simulink model "PID_centerlineTracking"  (R2023b)
settings: Solver=VariableStepAuto  StartTime=0.0  StopTime=Te  RelTol=1e-3
values from neighbouring files (symbols this model uses):
  Ts = 0.1    [ScriptBoot.m]    (also in ScriptBoot_TEST.m)
undefined symbols (not defined in the file or in its folder): accMAX, brakeMAX, driving, egoCarID, jerkMAX, lr, m, position0, turnAngleMAX, turnAngleRateMAX, velocity0
libraries: drivingscenarioandsensors x7, robotcorelib x2, autolibshared x1, sensorinslib x1
(part 1 of 3)
settings Model: Creator=Victor  LastModifiedBy=Victor

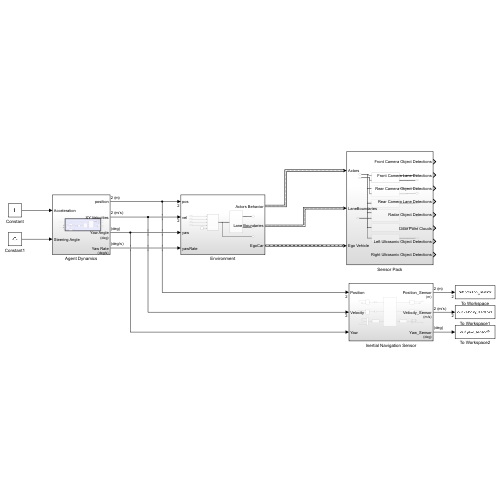
[thumbnail: Simulink's stored preview of the top-level diagram]
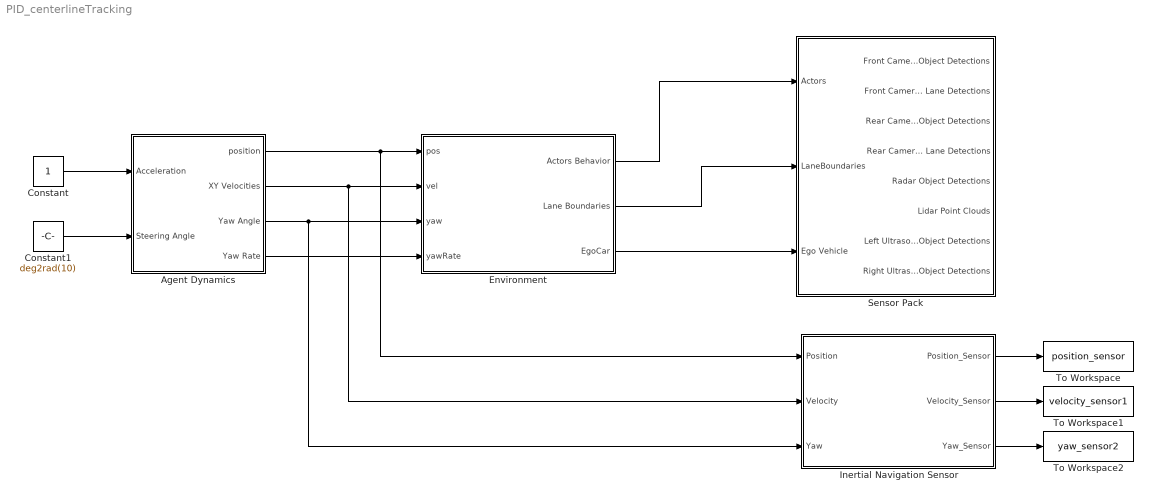
== system PID_centerlineTracking ==
  Agent Dynamics : Subsystem
  Constant : Constant
  Constant1 : Constant  Value=deg2rad(10)
  Environment : Subsystem
  Inertial Navigation Sensor : Subsystem
  Sensor Pack : Subsystem
  To Workspace : ToWorkspace  VariableName=position_sensor  SaveFormat=Timeseries  SampleTime=-1
  To Workspace1 : ToWorkspace  VariableName=velocity_sensor1  SaveFormat=Timeseries  SampleTime=-1
  To Workspace2 : ToWorkspace  VariableName=yaw_sensor2  SaveFormat=Timeseries  SampleTime=-1
  wires:
  Constant/1 -> Agent Dynamics/1(Acceleration)
  Constant1/1 -> Agent Dynamics/2(Steering Angle)
  Agent Dynamics/1(position) -> Inertial Navigation Sensor/1(Position), Environment/1(pos)
  Agent Dynamics/2(XY Velocities) -> Inertial Navigation Sensor/2(Velocity), Environment/2(vel)
  Agent Dynamics/3(Yaw Angle) -> Inertial Navigation Sensor/3(Yaw), Environment/3(yaw)
  Agent Dynamics/4(Yaw Rate) -> Environment/4(yawRate)
  Inertial Navigation Sensor/3(Yaw_Sensor) -> To Workspace2/1
  Inertial Navigation Sensor/2(Velocity_Sensor) -> To Workspace1/1
  Inertial Navigation Sensor/1(Position_Sensor) -> To Workspace/1
  Environment/1(Actors Behavior) -> Sensor Pack/1(Actors)
  Environment/2(Lane Boundaries) -> Sensor Pack/2(LaneBoundaries)
  Environment/3(EgoCar) -> Sensor Pack/3(Ego Vehicle)

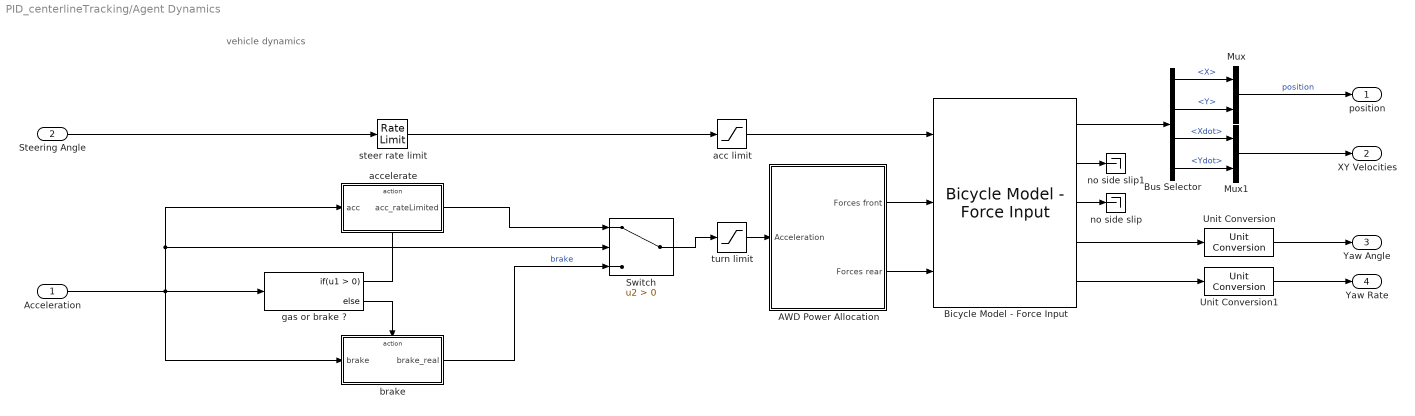
== system PID_centerlineTracking/Agent Dynamics ==
  note: vehicle dynamics
  Acceleration : Inport
  Steering Angle : Inport  Port=2
  AWD Power Allocation : Subsystem
  Bicycle Model - Force Input : autolibshared/Bicycle Model - Force Input  trackMode=Single (bicycle)  inputMode=External longitudinal forces  frontSteerMode=on  rearSteerMode=off  windMode=off  muMode=off  extFMode=off  extMMode=off  aMode=3  NF=2  NR=2  m=m  a=lf  b=lr  h=0.35  X_o=position0(1)  xdot_o=velocity0(1)  CalphaMode=off  sigmaMode=on  w=[1.4,1.4]  Cy_f=Cf  Cy_r=Cr  sigma_f=.1  sigma_r=.1  alpha_f_brk=[-.1 .1]  Cy_f_data=[-9e3 9e3]  alpha_r_brk=[-.1 .1]  Cy_r_data=[-9e3 9e3]  Y_o=position0(2)  ydot_o=velocity0(2)  Izz=Iz  psi_o=yaw0  r_o=yawRate0  Af=0  Cd=.3  Cl=.1  Cpm=.1  beta_w=[0:0.01:0.3]  Cs=[0:0.03:0.9]  Cym=[0:0.01:0.3]  Pabs=101325  Tair=273  g=9.81  mu=1  xdot_tol=.01  Fznom=5000  Fxtire_sat=1e6  Fytire_sat=1e6  longOff=0  latOff=0  vertOff=0
      settings: LibrarySourceBlock=drivingscenarioandsensors/Bicycle Model - Force Input
  Bus Selector : BusSelector  OutputSignals=InertFrm.FrntAxl.Disp.X,InertFrm.FrntAxl.Disp.Y,InertFrm.FrntAxl.Vel.Xdot,InertFrm.FrntAxl.Vel.Ydot
  Mux : Mux  Inputs=2
  Mux1 : Mux  Inputs=2
  Switch : Switch  Criteria=u2 > Threshold  SaturateOnIntegerOverflow=off  InputSameDT=off
  Unit Conversion : UnitConversion  OutputType=Inherit: Inherit via back propagation
  Unit Conversion1 : UnitConversion  OutputType=Inherit: Inherit via back propagation
  acc limit : Saturate  UpperLimit=accMAX  LowerLimit=-brakeMAX
  accelerate : Subsystem  TreatAsAtomicUnit=on
  brake : Subsystem  TreatAsAtomicUnit=on
  gas or brake ? : If
  no side slip : Terminator
  no side slip1 : Terminator
  steer rate limit : RateLimiter  RisingSlewLimit=turnAngleRateMAX  FallingSlewLimit=-turnAngleRateMAX  SampleTimeMode=inherited
  turn limit : Saturate  UpperLimit=turnAngleMAX  LowerLimit=-turnAngleMAX
  position : Outport
  XY Velocities : Outport  Port=2
  Yaw Angle : Outport  Port=3  Unit=deg
  Yaw Rate : Outport  Port=4  Unit=deg/s
  wires:
  Mux1/1 -> XY Velocities/1
  Unit Conversion/1 -> Yaw Angle/1
  Unit Conversion1/1 -> Yaw Rate/1
  accelerate/1(acc_rateLimited) -> Switch/1
  Steering Angle/1 -> steer rate limit/1
  acc limit/1 -> Bicycle Model - Force Input/1
  steer rate limit/1 -> acc limit/1
  Switch/1 -> turn limit/1
  turn limit/1 -> AWD Power Allocation/1(Acceleration)
  Bus Selector/2 -> Mux/2  "<Y>"
  Bus Selector/3 -> Mux1/1  "<Xdot>"
  Bicycle Model - Force Input/1 -> Bus Selector/1
  gas or brake ?/1 -> accelerate/Action
  Bus Selector/1 -> Mux/1  "<X>"
  AWD Power Allocation/2(Forces rear) -> Bicycle Model - Force Input/3
  Mux/1 -> position/1  "position"
  gas or brake ?/2 -> brake/Action
  Bicycle Model - Force Input/3 -> no side slip/1
  Bicycle Model - Force Input/5 -> Unit Conversion1/1
  Bicycle Model - Force Input/4 -> Unit Conversion/1
  Bus Selector/4 -> Mux1/2  "<Ydot>"
  Acceleration/1 -> brake/1(brake), accelerate/1(acc), Switch/2, gas or brake ?/1
  brake/1(brake_real) -> Switch/3  "brake"
  Bicycle Model - Force Input/2 -> no side slip1/1
  AWD Power Allocation/1(Forces front) -> Bicycle Model - Force Input/2

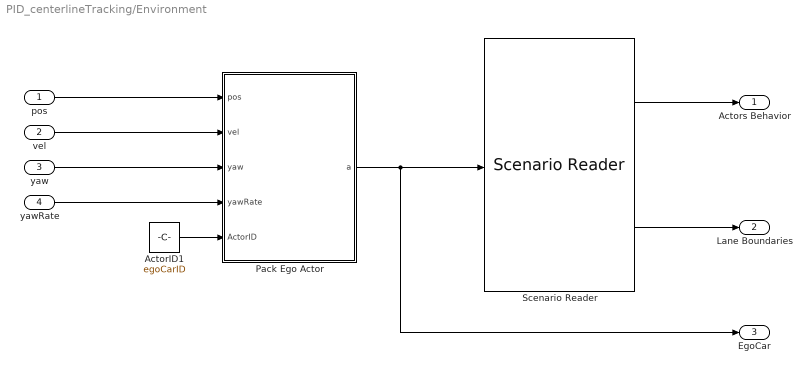
== system PID_centerlineTracking/Environment ==
  pos : Inport
  vel : Inport  Port=2
  yaw : Inport  Port=3
  yawRate : Inport  Port=4
  ActorID1 : Constant  Value=egoCarID
  Pack Ego Actor : MATLAB Function  TreatAsAtomicUnit=on
  Scenario Reader : drivingscenarioandsensors/Scenario Reader  ScenarioSource=From file  ScenarioFileName=Scenario_OneEgoCar.mat  ScenarioVariableName=scenario  OutputCoordinateSystem=Vehicle coordinates  EgoVehicleSource=Input port  EgoVehicleActorID=egoCarID  OrientVehiclesOnRoad=on  OutputEgoVehiclePose=off  OutputEgoVehicleState=off  SampleTime=Ts  LaneBoundaryOutput=Ego vehicle lane boundaries  LaneBoundaryDistance=0:0.5:60  LaneBoundaryLocation=Inner edge of lane markings  BusNameSource=Auto  BusName=BusActors  BusNumActorsSource=Scenario  BusNumActors=100  BusName2Source=Auto  BusName2=BusLaneBoundaries  BusNumLaneBoundariesSource=Scenario  BusNumLaneBoundaries=10  BusName3Source=Auto  BusName3=BusEgoActor  BusName4Source=Auto  BusName4=BusEgoState  ShowCoordinateLabels=on  SimulateUsing=Interpreted execution
  Actors Behavior : Outport
  Lane Boundaries : Outport  Port=2
  EgoCar : Outport  Port=3
  wires:
  pos/1 -> Pack Ego Actor/1(pos)
  Pack Ego Actor/1(a) -> Scenario Reader/1, EgoCar/1
  ActorID1/1 -> Pack Ego Actor/5(ActorID)
  Scenario Reader/1 -> Actors Behavior/1
  vel/1 -> Pack Ego Actor/2(vel)
  yaw/1 -> Pack Ego Actor/3(yaw)
  yawRate/1 -> Pack Ego Actor/4(yawRate)
  Scenario Reader/2 -> Lane Boundaries/1

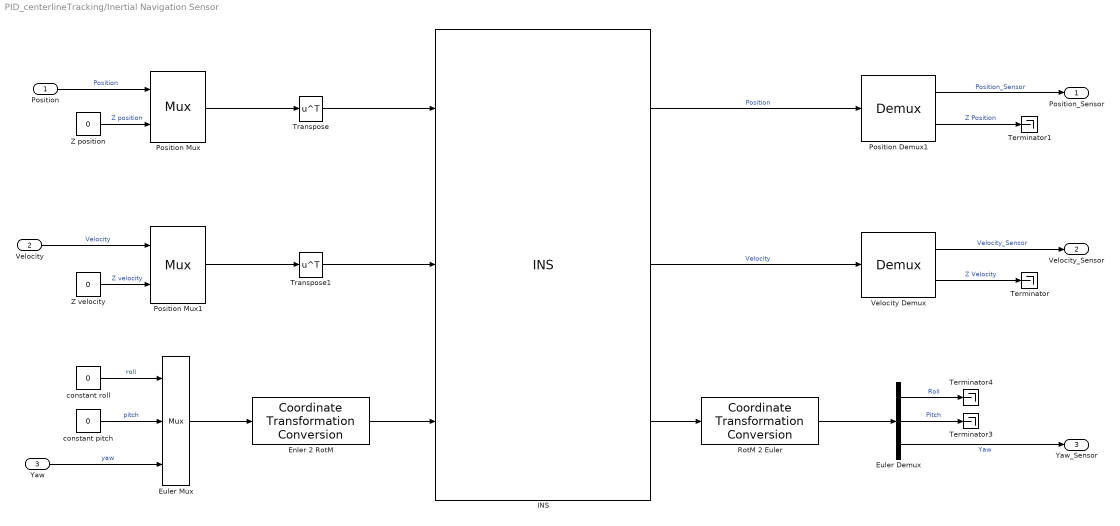
== system PID_centerlineTracking/Inertial Navigation Sensor ==
  Position : Inport
  Velocity : Inport  Port=2
  Yaw : Inport  Port=3
  Enler 2 RotM : robotcorelib/Coordinate Transformation Conversion  InputRepresentation=Euler Angles  InputEulerSequence=XYZ  ShowTrVecInputPort=on  OutputRepresentation=Rotation Matrix  OutputEulerSequence=XYZ  ShowTrVecOutputPort=on  SimulateUsing=Interpreted execution
      settings: LibrarySourceBlock=uavutilslib/Coordinate Transformation Conversion
  Euler Demux : Demux  Outputs=3
      settings: DisplayOption=none
  Euler Mux : Mux  Inputs=3
      settings: DisplayOption=signals
  INS : sensorinslib/INS  MountingLocation=[0 0 0]  RollAccuracy=angleAccuraccy  PitchAccuracy=angleAccuraccy  YawAccuracy=angleAccuraccy  PositionAccuracy=positionAccuracy  VelocityAccuracy=velocityAccuracy  UseAccelAndAngVel=off  AccelerationAccuracy=0  AngularVelocityAccuracy=0  TimeInput=off  PositionErrorFactor=[0 0 0]  SeedDouble=32  SimulateUsing=Interpreted execution
      settings: LibrarySourceBlock=drivingscenarioandsensors/INS
  Position Demux1 : Demux  Outputs=2
  Position Mux : Mux  Inputs=2
      settings: DisplayOption=signals
  Position Mux1 : Mux  Inputs=2
      settings: DisplayOption=signals
  RotM 2 Euler : robotcorelib/Coordinate Transformation Conversion  InputRepresentation=Rotation Matrix  InputEulerSequence=XYZ  ShowTrVecInputPort=on  OutputRepresentation=Euler Angles  OutputEulerSequence=XYZ  ShowTrVecOutputPort=on  SimulateUsing=Interpreted execution
      settings: LibrarySourceBlock=uavutilslib/Coordinate Transformation Conversion
  Terminator{,1,3..4} (4 alike) : Terminator
  Transpose : Math  Operator=transpose
  Transpose1 : Math  Operator=transpose
  Velocity Demux : Demux  Outputs=2
  Z position : Constant  Value=0
  Z velocity : Constant  Value=0
  constant pitch : Constant  Value=0
  constant roll : Constant  Value=0
  Position_Sensor : Outport  Unit=m  PortDimensions=2
  Velocity_Sensor : Outport  Port=2  Unit=m/s  PortDimensions=2
  Yaw_Sensor : Outport  Port=3  Unit=deg
  wires:
  Enler 2 RotM/1 -> INS/3
  Euler Demux/1 -> Terminator4/1  "Roll"
  Euler Mux/1 -> Enler 2 RotM/1
  RotM 2 Euler/1 -> Euler Demux/1
  Euler Demux/3 -> Yaw_Sensor/1  "Yaw"
  INS/3 -> RotM 2 Euler/1
  Euler Demux/2 -> Terminator3/1  "Pitch"
  constant roll/1 -> Euler Mux/1  "roll"
  constant pitch/1 -> Euler Mux/2  "pitch"
  Yaw/1 -> Euler Mux/3  "yaw"
  Position/1 -> Position Mux/1  "Position"
  Z position/1 -> Position Mux/2  "Z position"
  Z velocity/1 -> Position Mux1/2  "Z velocity"
  Velocity/1 -> Position Mux1/1  "Velocity"
  Position Mux/1 -> Transpose/1
  Transpose/1 -> INS/1
  Position Mux1/1 -> Transpose1/1
  Transpose1/1 -> INS/2
  INS/2 -> Velocity Demux/1  "Velocity"
  Velocity Demux/1 -> Velocity_Sensor/1  "Velocity_Sensor"
  Velocity Demux/2 -> Terminator/1  "Z Velocity"
  Position Demux1/1 -> Position_Sensor/1  "Position_Sensor"
  Position Demux1/2 -> Terminator1/1  "Z Position"
  INS/1 -> Position Demux1/1  "Position"
